simulink model "Continuo"  (Simulink 6.3)
settings: Solver=ode45  StartTime=0.0  StopTime=10  RelTol=1e-3
settings Model: LastModifiedBy=Frank Gloria  StrictBusMsg=None
settings OptimizationCC: InlineInvariantSignals=on

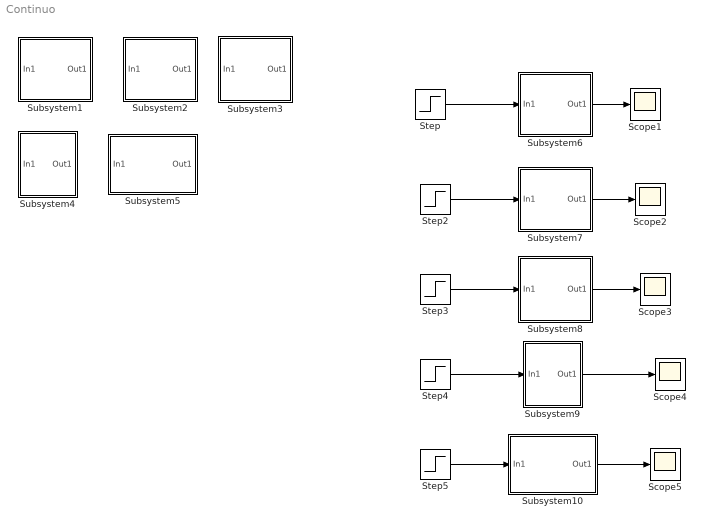
== system Continuo ==
  Scope{1..5} (5 alike) : Scope
      Scope3 settings: SaveName=ScopeData2
      Scope4 settings: SaveName=ScopeData3
      Scope5 settings: SaveName=ScopeData4
  Step{,2..5} (5 alike) : Step  Before=1  SampleTime=0
  "Subsystem1 " : Subsystem
      mask Display: disp('Planta P1')
  Subsystem10 : Subsystem
      mask Display: disp('Planta P5')
  Subsystem2 : Subsystem
      mask Display: disp('Planta P2')
  Subsystem3 : Subsystem
      mask Display: disp('Planta P3')
  Subsystem4 : Subsystem
      mask Display: disp('Planta P4')
  Subsystem5 : Subsystem
      mask Display: disp('Planta P5')
  Subsystem6 : Subsystem
      mask Display: disp('Planta P1')
  Subsystem7 : Subsystem
      mask Display: disp('Planta P2')
  Subsystem8 : Subsystem
      mask Display: disp('Planta P3')
  Subsystem9 : Subsystem
      mask Display: disp('Planta P4')
  wires:
  Step/1 -> Subsystem6/1(In1)
  Subsystem6/1(Out1) -> Scope1/1
  Step2/1 -> Subsystem7/1(In1)
  Step3/1 -> Subsystem8/1(In1)
  Step4/1 -> Subsystem9/1(In1)
  Step5/1 -> Subsystem10/1(In1)
  Subsystem10/1(Out1) -> Scope5/1
  Subsystem9/1(Out1) -> Scope4/1
  Subsystem8/1(Out1) -> Scope3/1
  Subsystem7/1(Out1) -> Scope2/1

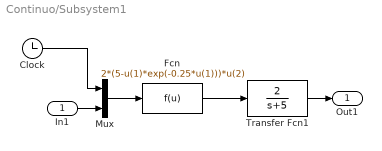
== system Continuo/Subsystem1  ==
  In1 : Inport
  Clock : Clock
      settings: Decimation=10
  Fcn : Fcn  Expr=2*(5-u(1)*exp(-0.25*u(1)))*u(2)
  Mux : Mux  Inputs=2
  Transfer Fcn1 : TransferFcn  Numerator=[2]  Denominator=[1 5]
  Out1 : Outport
  wires:
  Clock/1 -> Mux/1
  Mux/1 -> Fcn/1
  Fcn/1 -> Transfer Fcn1/1
  Transfer Fcn1/1 -> Out1/1
  In1/1 -> Mux/2

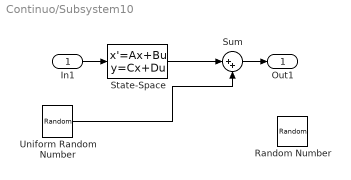
== system Continuo/Subsystem10 ==
  In1 : Inport
  Random Number : RandomNumber  Variance=0.25  SampleTime=0
  State-Space : StateSpace  A=[-1 -2;1 0]  B=[1; 0]  C="[0  2]"  D=0
  Sum : Sum  Inputs=|++
  Uniform Random Number : UniformRandomNumber  Minimum=-0.25  Maximum=0.25  SampleTime=0
  Out1 : Outport
  wires:
  State-Space/1 -> Sum/1
  In1/1 -> State-Space/1
  Sum/1 -> Out1/1
  Uniform Random Number/1 -> Sum/2

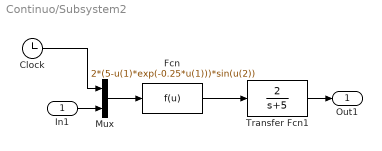
== system Continuo/Subsystem2 ==
  In1 : Inport
  Clock : Clock
      settings: Decimation=10
  Fcn : Fcn  Expr=2*(5-u(1)*exp(-0.25*u(1)))*sin(u(2))
  Mux : Mux  Inputs=2
  Transfer Fcn1 : TransferFcn  Numerator=[2]  Denominator=[1 5]
  Out1 : Outport
  wires:
  Clock/1 -> Mux/1
  Mux/1 -> Fcn/1
  Fcn/1 -> Transfer Fcn1/1
  Transfer Fcn1/1 -> Out1/1
  In1/1 -> Mux/2

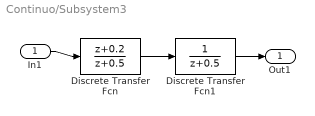
== system Continuo/Subsystem3 ==
  In1 : Inport
  Discrete Transfer Fcn : DiscreteTransferFcn  Numerator=[1 0.2]
  Discrete Transfer Fcn1 : DiscreteTransferFcn
  Out1 : Outport
  wires:
  Discrete Transfer Fcn/1 -> Discrete Transfer Fcn1/1
  Discrete Transfer Fcn1/1 -> Out1/1
  In1/1 -> Discrete Transfer Fcn/1

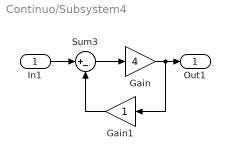
== system Continuo/Subsystem4 ==
  In1 : Inport
  Gain : Gain  Gain=4
  Gain1 : Gain  Orientation=left
  Sum3 : Sum  Inputs=|+-
  Out1 : Outport
  wires:
  Sum3/1 -> Gain/1
  Gain1/1 -> Sum3/2
  Gain/1 -> Out1/1, Gain1/1
  In1/1 -> Sum3/1

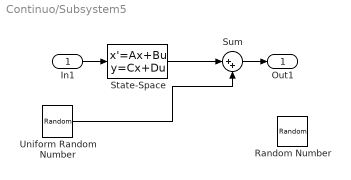
== system Continuo/Subsystem5 ==
  In1 : Inport
  Random Number : RandomNumber  Variance=0.25  SampleTime=0
  State-Space : StateSpace  A=[-1 -2;1 0]  B=[1; 0]  C="[0  2]"  D=0
  Sum : Sum  Inputs=|++
  Uniform Random Number : UniformRandomNumber  Minimum=-0.25  Maximum=0.25  SampleTime=0
  Out1 : Outport
  wires:
  State-Space/1 -> Sum/1
  In1/1 -> State-Space/1
  Sum/1 -> Out1/1
  Uniform Random Number/1 -> Sum/2

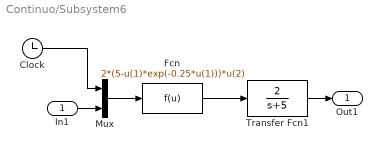
== system Continuo/Subsystem6 ==
  In1 : Inport
  Clock : Clock
      settings: Decimation=10
  Fcn : Fcn  Expr=2*(5-u(1)*exp(-0.25*u(1)))*u(2)
  Mux : Mux  Inputs=2
  Transfer Fcn1 : TransferFcn  Numerator=[2]  Denominator=[1 5]
  Out1 : Outport
  wires:
  Clock/1 -> Mux/1
  Mux/1 -> Fcn/1
  Fcn/1 -> Transfer Fcn1/1
  Transfer Fcn1/1 -> Out1/1
  In1/1 -> Mux/2

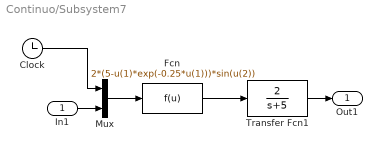
== system Continuo/Subsystem7 ==
  In1 : Inport
  Clock : Clock
      settings: Decimation=10
  Fcn : Fcn  Expr=2*(5-u(1)*exp(-0.25*u(1)))*sin(u(2))
  Mux : Mux  Inputs=2
  Transfer Fcn1 : TransferFcn  Numerator=[2]  Denominator=[1 5]
  Out1 : Outport
  wires:
  Clock/1 -> Mux/1
  Mux/1 -> Fcn/1
  Fcn/1 -> Transfer Fcn1/1
  Transfer Fcn1/1 -> Out1/1
  In1/1 -> Mux/2

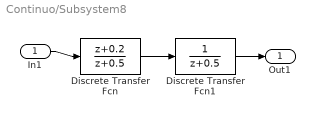
== system Continuo/Subsystem8 ==
  In1 : Inport
  Discrete Transfer Fcn : DiscreteTransferFcn  Numerator=[1 0.2]
  Discrete Transfer Fcn1 : DiscreteTransferFcn
  Out1 : Outport
  wires:
  Discrete Transfer Fcn/1 -> Discrete Transfer Fcn1/1
  Discrete Transfer Fcn1/1 -> Out1/1
  In1/1 -> Discrete Transfer Fcn/1

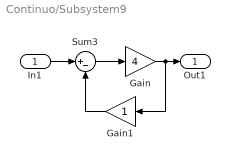
== system Continuo/Subsystem9 ==
  In1 : Inport
  Gain : Gain  Gain=4
  Gain1 : Gain  Orientation=left
  Sum3 : Sum  Inputs=|+-
  Out1 : Outport
  wires:
  Sum3/1 -> Gain/1
  Gain1/1 -> Sum3/2
  Gain/1 -> Out1/1, Gain1/1
  In1/1 -> Sum3/1
